simulink model "HarnessModel_RoadGradeProfile_CustomComponent"  (R2026a)
settings: Solver=VariableStepAuto  StopTime=1000
libraries: nesl_utility x3, fl_lib x1
settings Model: Creator=isaacito  LastModifiedBy=isaacito

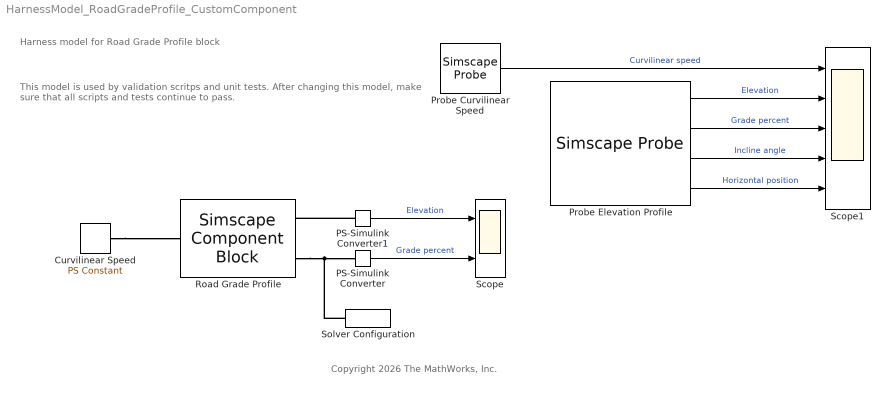
== system HarnessModel_RoadGradeProfile_CustomComponent ==
  note: This model is used by validation scritps and unit tests. After changing this model, make sure that all scripts and tests continue to pass.
  note: Harness model for Road Grade Profile block
  note: Copyright 2026 The MathWorks, Inc.
  Curvilinear Speed : fl_lib/Physical Signals/Sources/PS Constant  constant=1 m/s
      settings: AttributesFormatString=%<constant_unit>
  PS-Simulink Converter : nesl_utility/PS-Simulink Converter  PhysicalDomain=network_engine_domain  SubClassName=ps_output  LeftPortType=input  RightPortType=output  PseudoPeriodic=off  Frequencies=[]  VectorFormat=inherit  Unit=1  AffineConversion=off
  PS-Simulink Converter1 : nesl_utility/PS-Simulink Converter  PhysicalDomain=network_engine_domain  SubClassName=ps_output  LeftPortType=input  RightPortType=output  PseudoPeriodic=off  Frequencies=[]  VectorFormat=inherit  Unit=m  AffineConversion=off
  Probe Curvilinear Speed : SimscapeProbe  BoundBlock=2  Variables="{\"O\":{\"Probing\":\"ON\"}}"
  Probe Elevation Profile : SimscapeProbe  BoundBlock=1  Variables="{\"Vs\":{\"Probing\":\"OFF\"},\"elevation\":{\"Probing\":\"ON\"},\"grade_pct_x\":{\"Probing\":\"ON\"},\"incline_angle_x\":{\"Probing\":\"ON\"},\"x\":{\"Probing\":\"ON\"}}"
  Road Grade Profile : SimscapeComponentBlock  SourceFile=RoadGradeProfile  ComponentPath=RoadGradeProfile  ComponentVariants="[\"RoadGradeProfile\"]"  ComponentVariantNames="[\"RoadGradeProfile\"]"  ClassName=RoadGradeProfile  SchemaVersion=1  x_vector=[0, 50, 100] m  grade_vector=[0, 0, 0]  profile_interp_method=simscape.enum.interpolation.smooth  initial_position=0 m  initial_elevation=0 m
      settings: CopyFcn=simscape.sscblock.internal.componentBlockCallback(gcbh,'COPY')  PreCopyFcn=simscape.sscblock.internal.componentBlockCallback(gcbh,'PRECOPY')  PreDeleteFcn=simscape.sscblock.internal.componentBlockCallback(gcbh,'PREDELETE')
      mask Type: Road Grade Profile
  Scope : Scope  NumInputPorts=2
      settings: ActiveDisplayYMinimum=-1  ActiveDisplayYMaximum=1
  Scope1 : Scope  NumInputPorts=5
      settings: ActiveDisplayYMinimum=-1  ActiveDisplayYMaximum=1
  Solver Configuration : nesl_utility/Solver Configuration  PhysicalDomain=network_engine_domain  SubClassName=solver  LeftPortType=input  RightPortType=generic  Tones=[]  Harmonics=[]  SimulateNoise=off  Profile=off  UseLocalSampling=off  EnableSwitchedLinearOptims=on  FrequencyDomain=off  UseCCode=off  RelTol=0.001  AbsTol=0.001  MinStep=1e-09  ToWorkspace=off  RevertToSquareIcSolve=off  NumHomotopyIterations=100  PhasorMode=off  PhasorModeNumHarmonics=1  ConsistencySolver=NEWTON_XTOL_AFTER_FTOL  CanonicalOrdering=CANONICAL  OptimizeIntermediates=OPTIMIZED  IndexReductionMethod=DerivativeReplacement  DoDC=off  ResidualTolerance=1e-09  ConsistencyTolSource=GLOBAL  ConsistencyAbsTol=0.001  ConsistencyRelTol=0.001  ConsistencyTolFactor=0.001  UseLocalSolver=off  LocalSolverChoice=NE_BACKWARD_EULER_ADVANCER  ResolveIndetEquations=on  FunctionEvalNumThread=1  LocalSolverSampleTime=0.001  DoFixedCost=off  MaxNonlinIter=3  MaxModeIter=2  ComputeImpulses=off  ImpulseIterations=2  LinearAlgebra=auto  LinearAlgebraNumThread=0  EquationFormulation=NE_TIME_EF  DelaysMemoryBudget=1024  AutomaticFiltering=on  FilteringTimeConstant=0.001  PartitionStorageMethod=AS_NEEDED  PartitionMemoryBudget=1024  PartitionMethod=ROBUST  MultibodyUseLocalSolver=off  MultibodyLocalSolverChoice=ODE1  MultibodyLocalSolverSampleTime=0.001
      settings: AttributesFormatString=Local solver: %<UseLocalSolver>
  wires:
  PS-Simulink Converter/1 -> Scope/2  "Grade percent"
  PS-Simulink Converter1/1 -> Scope/1  "Elevation"
  Probe Curvilinear Speed/1 -> Scope1/1  "Curvilinear speed"
  Probe Elevation Profile/1 -> Scope1/2  "Elevation"
  Probe Elevation Profile/2 -> Scope1/3  "Grade percent"
  Probe Elevation Profile/3 -> Scope1/4  "Incline angle"
  Probe Elevation Profile/4 -> Scope1/5  "Horizontal position"
  connections:
  Curvilinear Speed/RConn1 -- Road Grade Profile/LConn1
  Road Grade Profile/RConn2 -- Solver Configuration/RConn1 -- PS-Simulink Converter/LConn1
  PS-Simulink Converter1/LConn1 -- Road Grade Profile/RConn1
